simulink model "exampleSamplingTheorem"  (R2017a)
settings: Solver=VariableStepAuto  StartTime=0.0  StopTime=8  RelTol=1e-3
values from neighbouring files (symbols this model uses):
  Fp = 44000    [script.m]
  Kl = -5.31*0.0001*Fp+3.6    (= -19.764)    [script.m]
  Kr = -5.31*0.0001*Fp+3.6    (= -19.764)    [script.m]
libraries: dsparch4 x2
settings Model: Creator=root  LastModifiedBy=kenpachi

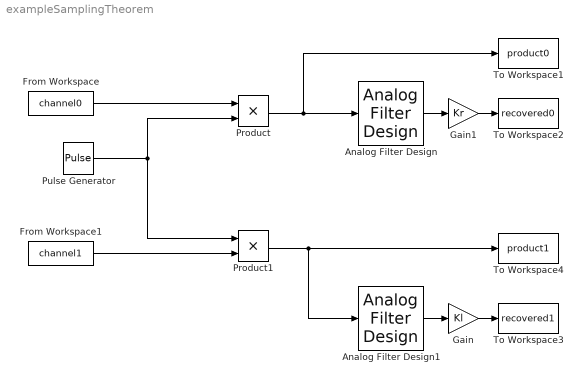
== system exampleSamplingTheorem ==
  Analog Filter Design : dsparch4/Analog Filter Design  method=Bessel  filttype=Lowpass  N=3  Wlo=2*pi*10000  Whi=80  Rp=2  Rs=40
  Analog Filter Design1 : dsparch4/Analog Filter Design  method=Bessel  filttype=Lowpass  N=3  Wlo=2*pi*10000  Whi=80  Rp=2  Rs=40
  From Workspace : FromWorkspace  VariableName=channel0  SampleTime=1/44100
  From Workspace1 : FromWorkspace  VariableName=channel1  SampleTime=1/44100
  Gain : Gain  Gain=Kl
  Gain1 : Gain  Gain=Kr
  Product : Product
  Product1 : Product
  Pulse Generator : DiscretePulseGenerator  PulseType=Time based  Period=1/Fp  PulseWidth=5
  To Workspace1 : ToWorkspace  VariableName=product0  SaveFormat=Timeseries  SampleTime=-1
  To Workspace2 : ToWorkspace  VariableName=recovered0  SaveFormat=Timeseries  SampleTime=1/44100
  To Workspace3 : ToWorkspace  VariableName=recovered1  SaveFormat=Timeseries  SampleTime=1/44100
  To Workspace4 : ToWorkspace  VariableName=product1  SaveFormat=Timeseries  SampleTime=-1
  wires:
  Pulse Generator/1 -> Product1/1, Product/2
  Analog Filter Design/1 -> Gain1/1
  From Workspace/1 -> Product/1
  From Workspace1/1 -> Product1/2
  Analog Filter Design1/1 -> Gain/1
  Gain1/1 -> To Workspace2/1
  Gain/1 -> To Workspace3/1
  Product/1 -> To Workspace1/1, Analog Filter Design/1
  Product1/1 -> To Workspace4/1, Analog Filter Design1/1
